simulink model "MCSI_simulation_2024_9_mod"  (R2021a)
settings: Solver=VariableStepAuto  StartTime=0.0  StopTime=5/cfg.fl  RelTol=1e-3
undefined symbols (not defined in the file or in its folder): cfg
libraries: spsIdealSwitchLib x54, spsSeriesRLCBranchLib x19, simulink x12, spsCurrentMeasurementLib x10, commutil2 x9, spsTriangleGeneratorLib x9, spsMeanLib x2, spsThreePhaseSeriesRLCBranchLib x2, spsThreePhaseVIMeasurementLib x2, spsControlledCurrentSourceLib x1, spsGroundLib x1, spsThreePhaseProgrammableGeneratorLib x1
settings Model: Creator=Damian  LastModifiedBy=Damian

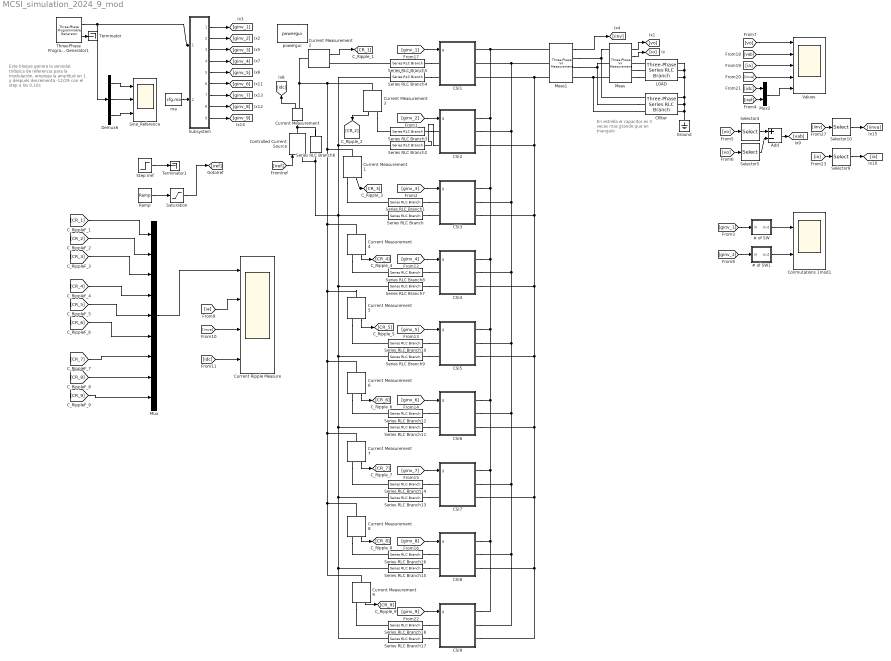
== system MCSI_simulation_2024_9_mod ==
  note: Este bloque genera la senoidal
      | trifásica de referencia para la
      | modulación, empieza la amplitud
      | en 1 y después decrementa -12/29
      | con el step a los 0.16s
  note: En estrella el capacitor
      | es 3 veces mas grande
      | que en triangulo
  # of SW : Subsystem
  # of SW1 : Subsystem
  Add : Sum  Inputs=+-
  CSI1 : Subsystem
  CSI2 : Subsystem
  CSI3 : Subsystem
  CSI4 : Subsystem
  CSI5 : Subsystem
  CSI6 : Subsystem
  CSI7 : Subsystem
  CSI8 : Subsystem
  CSI9 : Subsystem
  Cfilter : spsThreePhaseSeriesRLCBranchLib/Three-Phase Series RLC Branch  LConnTagsString=A|B|C  RConnTagsString=A|B|C  BranchType=C  Resistance=1  Inductance=cfg.c  Capacitance=cfg.c  Measurements=None
  Conmutations 1mod1 : Scope  NumInputPorts=2
  Controlled Current Source : spsControlledCurrentSourceLib/Controlled Current Source  Initialize=on  Source_Type=AC  Amplitude=0  Phase=0  Frequency=0  Measurements=None
  Current Measurement{,1..9} (10 alike) : spsCurrentMeasurementLib/Current Measurement  PhasorSimulation=off  OutputType=Complex  PSBequivalent=0
  Current Ripple Measure : Scope  NumInputPorts=4
  Demux6 : Demux  Outputs=3
  Ground : spsGroundLib/Ground  LConnTagsString=a
  LOAD : spsThreePhaseSeriesRLCBranchLib/Three-Phase Series RLC Branch  LConnTagsString=A|B|C  RConnTagsString=A|B|C  BranchType=RL  Resistance=cfg.r  Inductance=cfg.l  Capacitance=1e-6  Measurements=None
  Meas : spsThreePhaseVIMeasurementLib/Three-Phase V-I Measurement  VoltageMeasurement=phase-to-ground  SetLabelV=off  LabelV=Vabc  Vpu=off  VpuLL=off  CurrentMeasurement=yes  SetLabelI=off  LabelI=Iabc  Ipu=off  Pbase=100e6  Vbase=500e3  OutputType=Complex  PhasorSimulation=off  PSBequivalent=0
  Meas1 : spsThreePhaseVIMeasurementLib/Three-Phase V-I Measurement  VoltageMeasurement=no  SetLabelV=off  LabelV=Vabc  Vpu=off  VpuLL=off  CurrentMeasurement=yes  SetLabelI=off  LabelI=Iabc  Ipu=off  Pbase=100e6  Vbase=500e3  OutputType=Complex  PhasorSimulation=off  PSBequivalent=0
  Mux : Mux  Inputs=9
  Mux2 : Mux  Inputs=2
  Ramp : simulink/Sources/Ramp  slope=cfg.iref/cfg.cs_soft_start_time  start=0  InitialOutput=0
  Saturation : Saturate  UpperLimit=10  LowerLimit=0
  Selector10 : Selector  InputPortWidth=3  IndexOptions=Index vector (dialog)  Indices=1  OutputSizes=1
  Selector4 : Selector  InputPortWidth=3  IndexOptions=Index vector (dialog)  Indices=1  OutputSizes=1
  Selector5 : Selector  InputPortWidth=3  IndexOptions=Index vector (dialog)  Indices=2  OutputSizes=1
  Selector9 : Selector  InputPortWidth=3  IndexOptions=Index vector (dialog)  Indices=1  OutputSizes=1
  Series RLC Branch{,1..5,7..18} (18 alike) : spsSeriesRLCBranchLib/Series RLC Branch  LConnTagsString=__new0  RConnTagsString=__new0  BranchType=L  Resistance=1  Inductance=cfg.sharing_L  SetiL0=off  InitialCurrent=0  Capacitance=1e-6  Setx0=off  InitialVoltage=0  Measurements=None
  Series RLC Branch6 : spsSeriesRLCBranchLib/Series RLC Branch  LConnTagsString=__new0  RConnTagsString=__new0  BranchType=R  Resistance=1E5  Inductance=cfg.sharing_L  SetiL0=off  InitialCurrent=0  Capacitance=1e-6  Setx0=off  InitialVoltage=0  Measurements=None
  Sine_Reference : Scope  NumInputPorts=3
  Step Iref : Step  Time=12/cfg.fl  Before=cfg.iref  After=0.6*cfg.iref  SampleTime=cfg.ts
  Subsystem : Subsystem
  Terminator : Terminator
  Terminator1 : Terminator
  Three-Phase Programmable Generator1 : spsThreePhaseProgrammableGeneratorLib/Three-Phase Programmable Generator  Par_Vps=[1,-30, cfg.fl]  VariationEntity=None  VariationType=Step  VariationStep=-12/29  VariationRate=10  VariationMag=0.3  VariationFreq=2  Par_Timing_Variation="[8/cfg.fl  10]"  SinglePhase=on  Yampli=[1 0.2 1.2 1.0]  Xtime=[0 0.1 0.15 0.2]  HarmonicGeneration=off  Par_HarmoA="[3  5  -25 0]"  Par_HarmoB="[5  10  35  2]"  Par_Timing_Harmo="[ 0.05  99]"  Ts=cfg.ts
      settings: SourceProductBaseCode=PS
  Values : Scope  NumInputPorts=5
  ma : Constant  Value=cfg.ma
  powergui : spspowerguiLib/powergui  Priority=1  SimulationMode=Discrete  SampleTime=cfg.ts  frequency=60  Iterations=50  frequencyindice=0  Pbase=100e6  ErrMax=1e-4  UnitsV=kV  UnitsW=MW  buscounter=0  FunctionMessages=off  echomessages=off  EnableUseOfTLC=off  CurrentSourceSwitches=off  DisableSnubberDevices=off  DisableRonSwitches=off  DisableVfSwitches=off  DisplayEquations=off  AutomaticDiscreteSolvers=off  SolverType=Backward Euler  Interpol=off  ExternalGateDelay=off  methode=off  Ts=0  x0status=blocks  SPID=off  SwTol=0  HookPort=off  NonlinearTolerance=1e-4  nMaxIteration=100  ContinueOnMaxIteration=off  RestoreLinks=warning  ResistiveCurrentMeasurement=off  Frange=[0:2:500]  Ylog=off  Xlog=on  ShowGrid=off  save=off  variable=ZData  structure=one_mod_model  ZoomFFT=off  StartTime=0.12  cycles=1  DisplayStyle=1  fundamental=50  FreqAxis=off  MaxFrequency=1000  frequencyindicesteady=1  RmsSteady=1  display=off
  wires:
  [iref] -> Controlled Current Source/1
  Current Measurement/1 -> [idc]
  ma/1 -> Subsystem/2(ma)
  Three-Phase Programmable Generator1/2 -> Terminator/1
  Three-Phase Programmable Generator1/1 -> Subsystem/1(Vabc), Demux6/1
  Demux6/3 -> Sine_Reference/3
  Demux6/2 -> Sine_Reference/2
  Demux6/1 -> Sine_Reference/1
  [ginv_1] -> CSI1/1(g)
  Meas/1 -> [vo]
  Meas/2 -> [io]
  Meas1/1 -> [iinv]
  [iref] -> Mux2/2
  [idc] -> Mux2/1
  Mux2/1 -> Values/5
  [vo] -> Values/1
  [iinva] -> Values/4
  [ia] -> Values/3
  [vab] -> Values/2
  [vo] -> Selector4/1
  [vo] -> Selector5/1
  Selector4/1 -> Add/1
  Selector5/1 -> Add/2
  Add/1 -> [vab]
  [iinv] -> Selector10/1
  [io] -> Selector9/1
  Selector10/1 -> [iinva]
  Selector9/1 -> [ia]
  [ginv_2] -> CSI2/1(g)
  [ginv_3] -> CSI3/1(g)
  [ginv_1] -> # of SW/1(in)
  # of SW/1(out) -> Conmutations 1mod1/1
  # of SW1/1(out) -> Conmutations 1mod1/2
  [ginv_2] -> # of SW1/1(in)
  Saturation/1 -> [iref]
  Ramp/1 -> Saturation/1
  Step Iref/1 -> Terminator1/1
  Current Measurement2/1 -> [CR_1]
  Current Measurement3/1 -> [CR_2]
  Current Measurement1/1 -> [CR_3]
  [ia] -> Current Ripple Measure/2
  [iinva] -> Current Ripple Measure/3
  [idc] -> Current Ripple Measure/4
  [CR_1] -> Mux/1
  [CR_2] -> Mux/2
  [CR_3] -> Mux/3
  Mux/1 -> Current Ripple Measure/1
  Subsystem/1(g_1) -> [ginv_1]
  Subsystem/2(g_2) -> [ginv_2]
  Subsystem/3(g_3) -> [ginv_3]
  Subsystem/4(g_4) -> [ginv_4]
  Subsystem/5(g_5) -> [ginv_5]
  Subsystem/6(g_6) -> [ginv_6]
  Subsystem/7(g_7) -> [ginv_7]
  Subsystem/8(g_8) -> [ginv_8]
  Subsystem/9(g_9) -> [ginv_9]
  [ginv_4] -> CSI4/1(g)
  [ginv_5] -> CSI5/1(g)
  [ginv_6] -> CSI6/1(g)
  [ginv_7] -> CSI7/1(g)
  [ginv_8] -> CSI8/1(g)
  [ginv_9] -> CSI9/1(g)
  Current Measurement9/1 -> [CR_9]
  Current Measurement8/1 -> [CR_8]
  Current Measurement7/1 -> [CR_7]
  Current Measurement6/1 -> [CR_6]
  Current Measurement5/1 -> [CR_5]
  Current Measurement4/1 -> [CR_4]
  [CR_4] -> Mux/4
  [CR_5] -> Mux/5
  [CR_6] -> Mux/6
  [CR_7] -> Mux/7
  [CR_8] -> Mux/8
  [CR_9] -> Mux/9
  connections:
  Current Measurement/LConn1 -- Series RLC Branch6/LConn1 -- Controlled Current Source/RConn1
  Meas/LConn3 -- Cfilter/LConn3 -- Meas1/RConn3
  Meas/LConn1 -- Meas1/RConn1 -- Cfilter/LConn1
  LOAD/RConn2 -- LOAD/RConn1 -- LOAD/RConn3 -- Cfilter/RConn1 -- Cfilter/RConn2 -- Cfilter/RConn3 -- Ground/LConn1
  Cfilter/LConn2 -- Meas1/RConn2 -- Meas/LConn2
  LOAD/LConn1 -- Meas/RConn1
  Meas/RConn2 -- LOAD/LConn2
  Meas/RConn3 -- LOAD/LConn3
  Meas1/LConn1 -- CSI9/RConn1 -- CSI8/RConn1 -- CSI7/RConn1 -- CSI6/RConn1 -- CSI5/RConn1 -- CSI4/RConn1 -- CSI3/RConn1 -- CSI2/RConn1 -- CSI1/RConn1
  Meas1/LConn2 -- CSI9/RConn2 -- CSI8/RConn2 -- CSI7/RConn2 -- CSI6/RConn2 -- CSI5/RConn2 -- CSI4/RConn2 -- CSI3/RConn2 -- CSI2/RConn2 -- CSI1/RConn2
  Meas1/LConn3 -- CSI9/RConn3 -- CSI8/RConn3 -- CSI7/RConn3 -- CSI6/RConn3 -- CSI5/RConn3 -- CSI4/RConn3 -- CSI3/RConn3 -- CSI2/RConn3 -- CSI1/RConn3
  Series RLC Branch4/RConn1 -- CSI1/LConn2
  Series RLC Branch5/RConn1 -- CSI1/LConn1
  Series RLC Branch3/RConn1 -- CSI2/LConn2
  Series RLC Branch2/RConn1 -- CSI2/LConn1
  Series RLC Branch1/RConn1 -- CSI3/LConn1
  Series RLC Branch/RConn1 -- CSI3/LConn2
  Controlled Current Source/LConn1 -- Series RLC Branch17/LConn1 -- Series RLC Branch15/LConn1 -- Series RLC Branch13/LConn1 -- Series RLC Branch11/LConn1 -- Series RLC Branch9/LConn1 -- Series RLC Branch7/LConn1 -- Series RLC Branch2/LConn1 -- Series RLC Branch4/LConn1 -- Series RLC Branch/LConn1 -- Series RLC Branch6/RConn1
  Current Measurement3/RConn1 -- Series RLC Branch3/LConn1
  Current Measurement2/LConn1 -- Current Measurement1/LConn1 -- Current Measurement4/LConn1 -- Current Measurement5/LConn1 -- Current Measurement6/LConn1 -- Current Measurement7/LConn1 -- Current Measurement8/LConn1 -- Current Measurement9/LConn1 -- Current Measurement3/LConn1 -- Current Measurement/RConn1
  Current Measurement1/RConn1 -- Series RLC Branch1/LConn1
  Series RLC Branch5/LConn1 -- Current Measurement2/RConn1
  Series RLC Branch8/RConn1 -- CSI4/LConn1
  Series RLC Branch7/RConn1 -- CSI4/LConn2
  Series RLC Branch10/RConn1 -- CSI5/LConn1
  Series RLC Branch9/RConn1 -- CSI5/LConn2
  Series RLC Branch12/RConn1 -- CSI6/LConn1
  Series RLC Branch11/RConn1 -- CSI6/LConn2
  Series RLC Branch14/RConn1 -- CSI7/LConn1
  Series RLC Branch13/RConn1 -- CSI7/LConn2
  Series RLC Branch16/RConn1 -- CSI8/LConn1
  Series RLC Branch15/RConn1 -- CSI8/LConn2
  Series RLC Branch18/RConn1 -- CSI9/LConn1
  Series RLC Branch17/RConn1 -- CSI9/LConn2
  Current Measurement9/RConn1 -- Series RLC Branch18/LConn1
  Current Measurement8/RConn1 -- Series RLC Branch16/LConn1
  Current Measurement7/RConn1 -- Series RLC Branch14/LConn1
  Current Measurement6/RConn1 -- Series RLC Branch12/LConn1
  Current Measurement5/RConn1 -- Series RLC Branch10/LConn1
  Current Measurement4/RConn1 -- Series RLC Branch8/LConn1

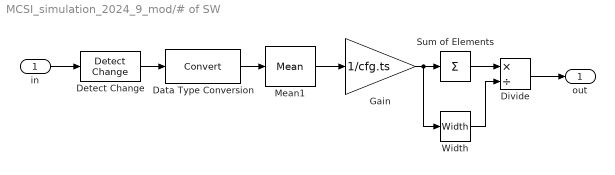
== system MCSI_simulation_2024_9_mod/# of SW ==
  in : Inport
  Data Type Conversion : DataTypeConversion
  Detect Change : simulink/Logic and Bit Operations/Detect Change  vinit=0  OutDataTypeStr=boolean
  Divide : Product  Inputs=*/
  Gain : Gain  Gain=1/cfg.ts
  Mean1 : spsMeanLib/Mean  Freq=cfg.fl  Vinit=0  Ts=cfg.ts
  Sum of Elements : Sum  Inputs=+
  Width : Width
  out : Outport
  wires:
  Detect Change/1 -> Data Type Conversion/1
  Mean1/1 -> Gain/1
  Data Type Conversion/1 -> Mean1/1
  in/1 -> Detect Change/1
  Gain/1 -> Width/1, Sum of Elements/1
  Sum of Elements/1 -> Divide/1
  Width/1 -> Divide/2
  Divide/1 -> out/1

== system MCSI_simulation_2024_9_mod/# of SW1 ==
  in : Inport
  Data Type Conversion : DataTypeConversion
  Detect Change : simulink/Logic and Bit Operations/Detect Change  vinit=0  OutDataTypeStr=boolean
  Gain : Gain  Gain=1/cfg.ts
  Mean1 : spsMeanLib/Mean  Freq=cfg.fl  Vinit=0  Ts=cfg.ts
  out : Outport
  wires:
  Detect Change/1 -> Data Type Conversion/1
  Mean1/1 -> Gain/1
  Data Type Conversion/1 -> Mean1/1
  in/1 -> Detect Change/1
  Gain/1 -> out/1

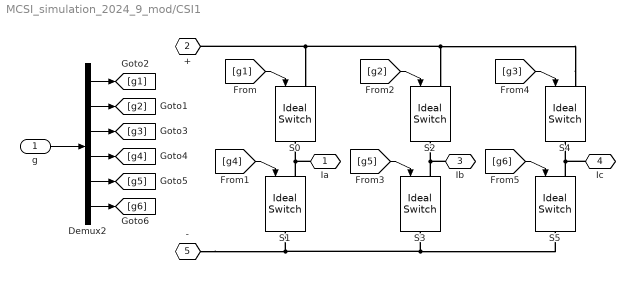
== system MCSI_simulation_2024_9_mod/CSI1 ==
  g : Inport
  Demux2 : Demux  Outputs=6
  S{0..5} (6 alike) : spsIdealSwitchLib/Ideal Switch  Ron=cfg.switch.Ron  Lon=0  IC=0  Rs=cfg.switch.snubber_Rs  Cs=cfg.switch.snubber_Cs  Measurements=off
  Ia : PMIOPort  Side=Right
  + : PMIOPort  Port=2  Side=Left
  Ib : PMIOPort  Port=3  Side=Right
  Ic : PMIOPort  Port=4  Side=Right
  - : PMIOPort  Port=5  Side=Left
  wires:
  Demux2/1 -> [g1]
  Demux2/4 -> [g4]
  g/1 -> Demux2/1
  [g4] -> S1/1
  [g2] -> S2/1
  [g5] -> S3/1
  Demux2/5 -> [g5]
  [g3] -> S4/1
  [g6] -> S5/1
  Demux2/6 -> [g6]
  Demux2/3 -> [g3]
  Demux2/2 -> [g2]
  [g1] -> S0/1
  connections:
  S1/LConn1 -- Ia/RConn1 -- S0/RConn1
  S3/LConn1 -- Ib/RConn1 -- S2/RConn1
  S5/LConn1 -- Ic/RConn1 -- S4/RConn1
  S4/LConn1 -- S2/LConn1 -- S0/LConn1 -- +/RConn1
  -/RConn1 -- S5/RConn1 -- S3/RConn1 -- S1/RConn1

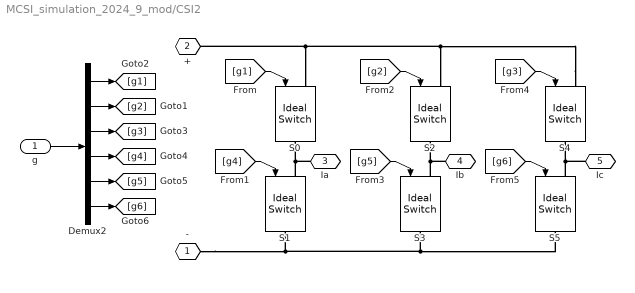
== system MCSI_simulation_2024_9_mod/CSI2 ==
  g : Inport
  Demux2 : Demux  Outputs=6
  S{0..5} (6 alike) : spsIdealSwitchLib/Ideal Switch  Ron=cfg.switch.Ron  Lon=0  IC=0  Rs=cfg.switch.snubber_Rs  Cs=cfg.switch.snubber_Cs  Measurements=off
  - : PMIOPort  Side=Left
  + : PMIOPort  Port=2  Side=Left
  Ia : PMIOPort  Port=3  Side=Right
  Ib : PMIOPort  Port=4  Side=Right
  Ic : PMIOPort  Port=5  Side=Right
  wires:
  Demux2/1 -> [g1]
  Demux2/4 -> [g4]
  g/1 -> Demux2/1
  [g4] -> S1/1
  [g2] -> S2/1
  [g5] -> S3/1
  Demux2/5 -> [g5]
  [g3] -> S4/1
  [g6] -> S5/1
  Demux2/6 -> [g6]
  Demux2/3 -> [g3]
  Demux2/2 -> [g2]
  [g1] -> S0/1
  connections:
  S1/LConn1 -- Ia/RConn1 -- S0/RConn1
  S3/LConn1 -- Ib/RConn1 -- S2/RConn1
  S5/LConn1 -- Ic/RConn1 -- S4/RConn1
  S4/LConn1 -- S2/LConn1 -- S0/LConn1 -- +/RConn1
  -/RConn1 -- S5/RConn1 -- S3/RConn1 -- S1/RConn1

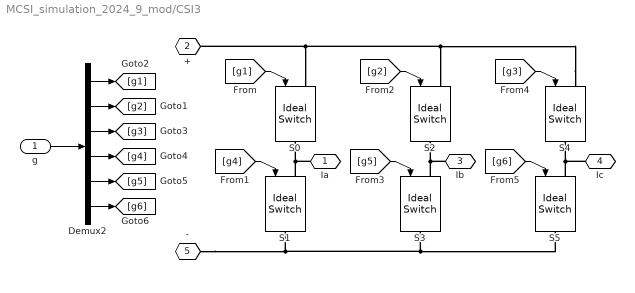
== system MCSI_simulation_2024_9_mod/CSI3 ==
  g : Inport
  Demux2 : Demux  Outputs=6
  S{0..5} (6 alike) : spsIdealSwitchLib/Ideal Switch  Ron=cfg.switch.Ron  Lon=0  IC=0  Rs=cfg.switch.snubber_Rs  Cs=cfg.switch.snubber_Cs  Measurements=off
  Ia : PMIOPort  Side=Right
  + : PMIOPort  Port=2  Side=Left
  Ib : PMIOPort  Port=3  Side=Right
  Ic : PMIOPort  Port=4  Side=Right
  - : PMIOPort  Port=5  Side=Left
  wires:
  Demux2/1 -> [g1]
  Demux2/4 -> [g4]
  g/1 -> Demux2/1
  [g4] -> S1/1
  [g2] -> S2/1
  [g5] -> S3/1
  Demux2/5 -> [g5]
  [g3] -> S4/1
  [g6] -> S5/1
  Demux2/6 -> [g6]
  Demux2/3 -> [g3]
  Demux2/2 -> [g2]
  [g1] -> S0/1
  connections:
  S1/LConn1 -- Ia/RConn1 -- S0/RConn1
  S3/LConn1 -- Ib/RConn1 -- S2/RConn1
  S5/LConn1 -- Ic/RConn1 -- S4/RConn1
  S4/LConn1 -- S2/LConn1 -- S0/LConn1 -- +/RConn1
  -/RConn1 -- S5/RConn1 -- S3/RConn1 -- S1/RConn1

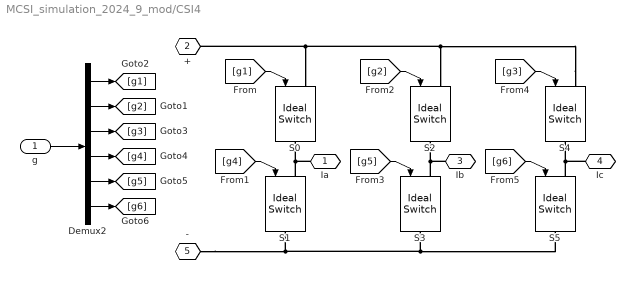
== system MCSI_simulation_2024_9_mod/CSI4 ==
  g : Inport
  Demux2 : Demux  Outputs=6
  S{0..5} (6 alike) : spsIdealSwitchLib/Ideal Switch  Ron=cfg.switch.Ron  Lon=0  IC=0  Rs=cfg.switch.snubber_Rs  Cs=cfg.switch.snubber_Cs  Measurements=off
  Ia : PMIOPort  Side=Right
  + : PMIOPort  Port=2  Side=Left
  Ib : PMIOPort  Port=3  Side=Right
  Ic : PMIOPort  Port=4  Side=Right
  - : PMIOPort  Port=5  Side=Left
  wires:
  Demux2/1 -> [g1]
  Demux2/4 -> [g4]
  g/1 -> Demux2/1
  [g4] -> S1/1
  [g2] -> S2/1
  [g5] -> S3/1
  Demux2/5 -> [g5]
  [g3] -> S4/1
  [g6] -> S5/1
  Demux2/6 -> [g6]
  Demux2/3 -> [g3]
  Demux2/2 -> [g2]
  [g1] -> S0/1
  connections:
  S1/LConn1 -- Ia/RConn1 -- S0/RConn1
  S3/LConn1 -- Ib/RConn1 -- S2/RConn1
  S5/LConn1 -- Ic/RConn1 -- S4/RConn1
  S4/LConn1 -- S2/LConn1 -- S0/LConn1 -- +/RConn1
  -/RConn1 -- S5/RConn1 -- S3/RConn1 -- S1/RConn1

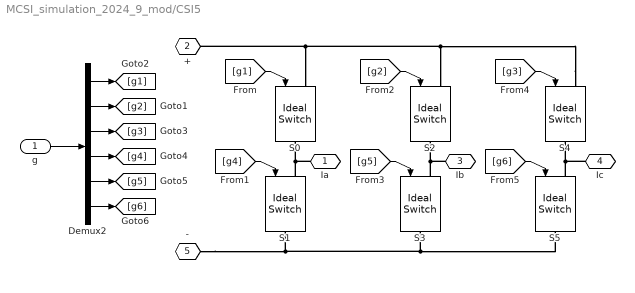
== system MCSI_simulation_2024_9_mod/CSI5 ==
  g : Inport
  Demux2 : Demux  Outputs=6
  S{0..5} (6 alike) : spsIdealSwitchLib/Ideal Switch  Ron=cfg.switch.Ron  Lon=0  IC=0  Rs=cfg.switch.snubber_Rs  Cs=cfg.switch.snubber_Cs  Measurements=off
  Ia : PMIOPort  Side=Right
  + : PMIOPort  Port=2  Side=Left
  Ib : PMIOPort  Port=3  Side=Right
  Ic : PMIOPort  Port=4  Side=Right
  - : PMIOPort  Port=5  Side=Left
  wires:
  Demux2/1 -> [g1]
  Demux2/4 -> [g4]
  g/1 -> Demux2/1
  [g4] -> S1/1
  [g2] -> S2/1
  [g5] -> S3/1
  Demux2/5 -> [g5]
  [g3] -> S4/1
  [g6] -> S5/1
  Demux2/6 -> [g6]
  Demux2/3 -> [g3]
  Demux2/2 -> [g2]
  [g1] -> S0/1
  connections:
  S1/LConn1 -- Ia/RConn1 -- S0/RConn1
  S3/LConn1 -- Ib/RConn1 -- S2/RConn1
  S5/LConn1 -- Ic/RConn1 -- S4/RConn1
  S4/LConn1 -- S2/LConn1 -- S0/LConn1 -- +/RConn1
  -/RConn1 -- S5/RConn1 -- S3/RConn1 -- S1/RConn1

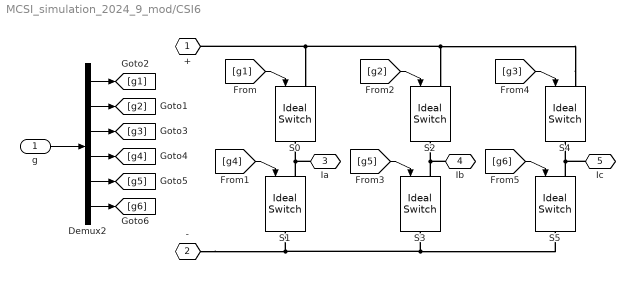
== system MCSI_simulation_2024_9_mod/CSI6 ==
  g : Inport
  Demux2 : Demux  Outputs=6
  S{0..5} (6 alike) : spsIdealSwitchLib/Ideal Switch  Ron=cfg.switch.Ron  Lon=0  IC=0  Rs=cfg.switch.snubber_Rs  Cs=cfg.switch.snubber_Cs  Measurements=off
  + : PMIOPort  Side=Left
  - : PMIOPort  Port=2  Side=Left
  Ia : PMIOPort  Port=3  Side=Right
  Ib : PMIOPort  Port=4  Side=Right
  Ic : PMIOPort  Port=5  Side=Right
  wires:
  Demux2/1 -> [g1]
  Demux2/4 -> [g4]
  g/1 -> Demux2/1
  [g4] -> S1/1
  [g2] -> S2/1
  [g5] -> S3/1
  Demux2/5 -> [g5]
  [g3] -> S4/1
  [g6] -> S5/1
  Demux2/6 -> [g6]
  Demux2/3 -> [g3]
  Demux2/2 -> [g2]
  [g1] -> S0/1
  connections:
  S1/LConn1 -- Ia/RConn1 -- S0/RConn1
  S3/LConn1 -- Ib/RConn1 -- S2/RConn1
  S5/LConn1 -- Ic/RConn1 -- S4/RConn1
  S4/LConn1 -- S2/LConn1 -- S0/LConn1 -- +/RConn1
  -/RConn1 -- S5/RConn1 -- S3/RConn1 -- S1/RConn1

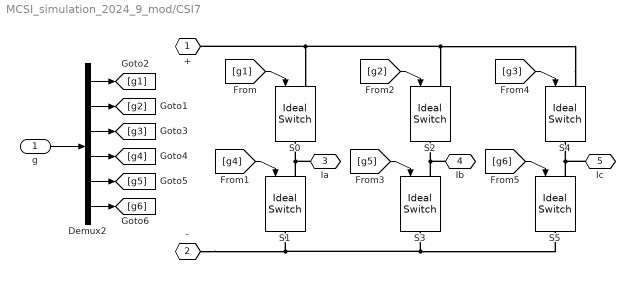
== system MCSI_simulation_2024_9_mod/CSI7 ==
  g : Inport
  Demux2 : Demux  Outputs=6
  S{0..5} (6 alike) : spsIdealSwitchLib/Ideal Switch  Ron=cfg.switch.Ron  Lon=0  IC=0  Rs=cfg.switch.snubber_Rs  Cs=cfg.switch.snubber_Cs  Measurements=off
  + : PMIOPort  Side=Left
  - : PMIOPort  Port=2  Side=Left
  Ia : PMIOPort  Port=3  Side=Right
  Ib : PMIOPort  Port=4  Side=Right
  Ic : PMIOPort  Port=5  Side=Right
  wires:
  Demux2/1 -> [g1]
  Demux2/4 -> [g4]
  g/1 -> Demux2/1
  [g4] -> S1/1
  [g2] -> S2/1
  [g5] -> S3/1
  Demux2/5 -> [g5]
  [g3] -> S4/1
  [g6] -> S5/1
  Demux2/6 -> [g6]
  Demux2/3 -> [g3]
  Demux2/2 -> [g2]
  [g1] -> S0/1
  connections:
  S1/LConn1 -- Ia/RConn1 -- S0/RConn1
  S3/LConn1 -- Ib/RConn1 -- S2/RConn1
  S5/LConn1 -- Ic/RConn1 -- S4/RConn1
  S4/LConn1 -- S2/LConn1 -- S0/LConn1 -- +/RConn1
  -/RConn1 -- S5/RConn1 -- S3/RConn1 -- S1/RConn1

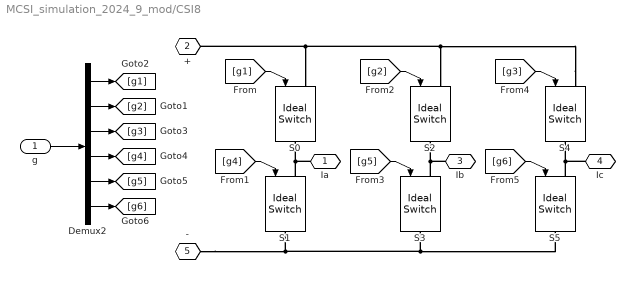
== system MCSI_simulation_2024_9_mod/CSI8 ==
  g : Inport
  Demux2 : Demux  Outputs=6
  S{0..5} (6 alike) : spsIdealSwitchLib/Ideal Switch  Ron=cfg.switch.Ron  Lon=0  IC=0  Rs=cfg.switch.snubber_Rs  Cs=cfg.switch.snubber_Cs  Measurements=off
  Ia : PMIOPort  Side=Right
  + : PMIOPort  Port=2  Side=Left
  Ib : PMIOPort  Port=3  Side=Right
  Ic : PMIOPort  Port=4  Side=Right
  - : PMIOPort  Port=5  Side=Left
  wires:
  Demux2/1 -> [g1]
  Demux2/4 -> [g4]
  g/1 -> Demux2/1
  [g4] -> S1/1
  [g2] -> S2/1
  [g5] -> S3/1
  Demux2/5 -> [g5]
  [g3] -> S4/1
  [g6] -> S5/1
  Demux2/6 -> [g6]
  Demux2/3 -> [g3]
  Demux2/2 -> [g2]
  [g1] -> S0/1
  connections:
  S1/LConn1 -- Ia/RConn1 -- S0/RConn1
  S3/LConn1 -- Ib/RConn1 -- S2/RConn1
  S5/LConn1 -- Ic/RConn1 -- S4/RConn1
  S4/LConn1 -- S2/LConn1 -- S0/LConn1 -- +/RConn1
  -/RConn1 -- S5/RConn1 -- S3/RConn1 -- S1/RConn1

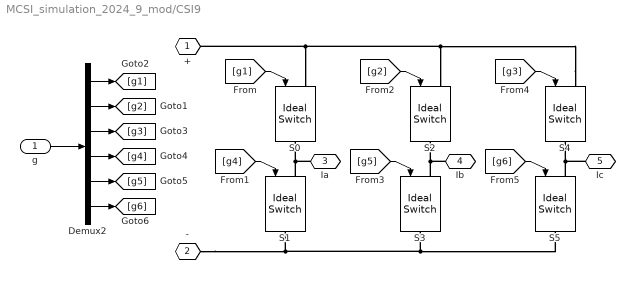
== system MCSI_simulation_2024_9_mod/CSI9 ==
  g : Inport
  Demux2 : Demux  Outputs=6
  S{0..5} (6 alike) : spsIdealSwitchLib/Ideal Switch  Ron=cfg.switch.Ron  Lon=0  IC=0  Rs=cfg.switch.snubber_Rs  Cs=cfg.switch.snubber_Cs  Measurements=off
  + : PMIOPort  Side=Left
  - : PMIOPort  Port=2  Side=Left
  Ia : PMIOPort  Port=3  Side=Right
  Ib : PMIOPort  Port=4  Side=Right
  Ic : PMIOPort  Port=5  Side=Right
  wires:
  Demux2/1 -> [g1]
  Demux2/4 -> [g4]
  g/1 -> Demux2/1
  [g4] -> S1/1
  [g2] -> S2/1
  [g5] -> S3/1
  Demux2/5 -> [g5]
  [g3] -> S4/1
  [g6] -> S5/1
  Demux2/6 -> [g6]
  Demux2/3 -> [g3]
  Demux2/2 -> [g2]
  [g1] -> S0/1
  connections:
  S1/LConn1 -- Ia/RConn1 -- S0/RConn1
  S3/LConn1 -- Ib/RConn1 -- S2/RConn1
  S5/LConn1 -- Ic/RConn1 -- S4/RConn1
  S4/LConn1 -- S2/LConn1 -- S0/LConn1 -- +/RConn1
  -/RConn1 -- S5/RConn1 -- S3/RConn1 -- S1/RConn1

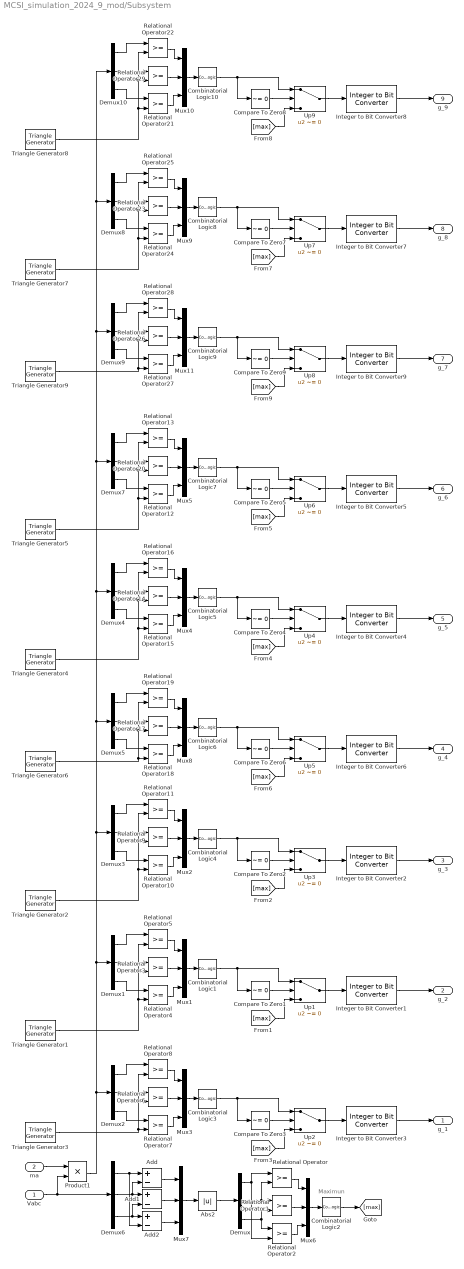
== system MCSI_simulation_2024_9_mod/Subsystem ==
  note: Maximun
  Vabc : Inport
  ma : Inport  Port=2
  Abs2 : Abs
  Add : Sum  Inputs=+-
  Add1 : Sum  Inputs=+-
  Add2 : Sum  Inputs=+-
  Combinatorial Logic{1,3..10} (9 alike) : CombinatorialLogic  TruthTable=bin2dec(['000000'; '001010'; '010100'; '001100'; '100001'; '100010'; '010001'; '000000'])
  Combinatorial Logic2 : CombinatorialLogic  TruthTable=bin2dec(['111111'; '001001'; '010010'; '010010'; '100100'; '001001'; '100100'; '111111'])
  Compare To Zero{1..9} (9 alike) : simulink/Logic and Bit Operations/Compare To Zero  relop=~=  OutDataTypeStr=boolean
  Demux{,1..10} (11 alike) : Demux  Outputs=3
  Integer to Bit Converter{1..9} (9 alike) : commutil2/Integer to Bit Converter  nbits=6  signedInputValues=Unsigned  bitOrder=MSB first  outDtype=Inherit via internal rule
  Mux{1..11} (11 alike) : Mux  Inputs=3
  Product1 : Product
  Relational Operator{,1..29} (30 alike) : RelationalOperator  OutDataTypeStr=boolean  RndMeth=Nearest
  Triangle Generator1 : spsTriangleGeneratorLib/Triangle Generator  Freq=cfg.fl*cfg.mf  Phase=1*cfg.tri_phase_shift  Ts=cfg.ts
  Triangle Generator2 : spsTriangleGeneratorLib/Triangle Generator  Freq=cfg.fl*cfg.mf  Phase=2*cfg.tri_phase_shift  Ts=cfg.ts
  Triangle Generator3 : spsTriangleGeneratorLib/Triangle Generator  Freq=cfg.fl*cfg.mf  Phase=0  Ts=cfg.ts
  Triangle Generator4 : spsTriangleGeneratorLib/Triangle Generator  Freq=cfg.fl*cfg.mf  Phase=4*cfg.tri_phase_shift  Ts=cfg.ts
  Triangle Generator5 : spsTriangleGeneratorLib/Triangle Generator  Freq=cfg.fl*cfg.mf  Phase=5*cfg.tri_phase_shift  Ts=cfg.ts
  Triangle Generator6 : spsTriangleGeneratorLib/Triangle Generator  Freq=cfg.fl*cfg.mf  Phase=3*cfg.tri_phase_shift  Ts=cfg.ts
  Triangle Generator7 : spsTriangleGeneratorLib/Triangle Generator  Freq=cfg.fl*cfg.mf  Phase=7*cfg.tri_phase_shift  Ts=cfg.ts
  Triangle Generator8 : spsTriangleGeneratorLib/Triangle Generator  Freq=cfg.fl*cfg.mf  Phase=8*cfg.tri_phase_shift  Ts=cfg.ts
  Triangle Generator9 : spsTriangleGeneratorLib/Triangle Generator  Freq=cfg.fl*cfg.mf  Phase=6*cfg.tri_phase_shift  Ts=cfg.ts
  Up{1..9} (9 alike) : Switch  Criteria=u2 ~= 0
  g_1 : Outport
  g_2 : Outport  Port=2
  g_3 : Outport  Port=3
  g_4 : Outport  Port=4
  g_5 : Outport  Port=5
  g_6 : Outport  Port=6
  g_7 : Outport  Port=7
  g_8 : Outport  Port=8
  g_9 : Outport  Port=9
  wires:
  Relational Operator/1 -> Mux6/1
  Demux/3 -> Relational Operator1/2, Relational Operator2/1
  Relational Operator1/1 -> Mux6/2
  Demux/2 -> Relational Operator/2, Relational Operator1/1
  Mux6/1 -> Combinatorial Logic2/1
  Relational Operator2/1 -> Mux6/3
  Vabc/1 -> Product1/2, Demux6/1
  Demux/1 -> Relational Operator/1, Relational Operator2/2
  Demux6/1 -> Add2/2, Add/1
  Demux6/2 -> Add/2, Add1/1
  Demux6/3 -> Add1/2, Add2/1
  Add/1 -> Mux7/1
  Add1/1 -> Mux7/2
  Add2/1 -> Mux7/3
  Abs2/1 -> Demux/1
  Mux7/1 -> Abs2/1
  Combinatorial Logic2/1 -> [max]
  ma/1 -> Product1/1
  Relational Operator7/1 -> Mux3/3
  Relational Operator8/1 -> Mux3/1
  Relational Operator6/1 -> Mux3/2
  Mux3/1 -> Combinatorial Logic3/1
  Combinatorial Logic3/1 -> Up2/1, Compare To Zero3/1
  Compare To Zero3/1 -> Up2/2
  Up2/1 -> Integer to Bit Converter3/1
  [max] -> Up2/3
  Triangle Generator3/1 -> Relational Operator8/2, Relational Operator6/2, Relational Operator7/2
  Demux2/3 -> Relational Operator7/1
  Demux2/2 -> Relational Operator6/1
  Demux2/1 -> Relational Operator8/1
  Integer to Bit Converter3/1 -> g_1/1
  Integer to Bit Converter1/1 -> g_2/1
  Relational Operator5/1 -> Mux1/1
  Demux1/1 -> Relational Operator5/1
  Mux1/1 -> Combinatorial Logic1/1
  Relational Operator3/1 -> Mux1/2
  [max] -> Up1/3
  Combinatorial Logic1/1 -> Up1/1, Compare To Zero1/1
  Demux1/2 -> Relational Operator3/1
  Up1/1 -> Integer to Bit Converter1/1
  Demux1/3 -> Relational Operator4/1
  Relational Operator4/1 -> Mux1/3
  Triangle Generator1/1 -> Relational Operator5/2, Relational Operator3/2, Relational Operator4/2
  Compare To Zero1/1 -> Up1/2
  Compare To Zero2/1 -> Up3/2
  Up3/1 -> Integer to Bit Converter2/1
  Relational Operator10/1 -> Mux2/3
  Demux3/2 -> Relational Operator9/1
  Demux3/3 -> Relational Operator10/1
  Relational Operator9/1 -> Mux2/2
  [max] -> Up3/3
  Demux3/1 -> Relational Operator11/1
  Combinatorial Logic4/1 -> Up3/1, Compare To Zero2/1
  Integer to Bit Converter2/1 -> g_3/1
  Relational Operator11/1 -> Mux2/1
  Triangle Generator2/1 -> Relational Operator11/2, Relational Operator9/2, Relational Operator10/2
  Mux2/1 -> Combinatorial Logic4/1
  Relational Operator13/1 -> Mux5/1
  Mux4/1 -> Combinatorial Logic5/1
  Integer to Bit Converter5/1 -> g_6/1
  Compare To Zero4/1 -> Up4/2
  Demux4/3 -> Relational Operator15/1
  Demux7/1 -> Relational Operator13/1
  Relational Operator15/1 -> Mux4/3
  Demux7/3 -> Relational Operator12/1
  [max] -> Up4/3
  Triangle Generator4/1 -> Relational Operator16/2, Relational Operator14/2, Relational Operator15/2
  Relational Operator20/1 -> Mux5/2
  Triangle Generator5/1 -> Relational Operator13/2, Relational Operator20/2, Relational Operator12/2
  Triangle Generator6/1 -> Relational Operator19/2, Relational Operator17/2, Relational Operator18/2
  Relational Operator19/1 -> Mux8/1
  Combinatorial Logic7/1 -> Up6/1, Compare To Zero5/1
  Combinatorial Logic6/1 -> Up5/1, Compare To Zero6/1
  Mux5/1 -> Combinatorial Logic7/1
  Mux8/1 -> Combinatorial Logic6/1
  [max] -> Up5/3
  Up5/1 -> Integer to Bit Converter6/1
  Demux7/2 -> Relational Operator20/1
  Integer to Bit Converter6/1 -> g_4/1
  Combinatorial Logic5/1 -> Up4/1, Compare To Zero4/1
  Compare To Zero5/1 -> Up6/2
  Up4/1 -> Integer to Bit Converter4/1
  Compare To Zero6/1 -> Up5/2
  Demux4/2 -> Relational Operator14/1
  Relational Operator14/1 -> Mux4/2
  [max] -> Up6/3
  Demux4/1 -> Relational Operator16/1
  Integer to Bit Converter4/1 -> g_5/1
  Relational Operator16/1 -> Mux4/1
  Demux5/1 -> Relational Operator19/1
  Demux5/2 -> Relational Operator17/1
  Relational Operator18/1 -> Mux8/3
  Relational Operator12/1 -> Mux5/3
  Demux5/3 -> Relational Operator18/1
  Relational Operator17/1 -> Mux8/2
  Up6/1 -> Integer to Bit Converter5/1
  Relational Operator22/1 -> Mux10/1
  Mux9/1 -> Combinatorial Logic8/1
  Integer to Bit Converter8/1 -> g_9/1
  Compare To Zero7/1 -> Up7/2
  Demux8/3 -> Relational Operator24/1
  Demux10/1 -> Relational Operator22/1
  Relational Operator24/1 -> Mux9/3
  Demux10/3 -> Relational Operator21/1
  [max] -> Up7/3
  Triangle Generator7/1 -> Relational Operator25/2, Relational Operator23/2, Relational Operator24/2
  Relational Operator29/1 -> Mux10/2
  Triangle Generator8/1 -> Relational Operator22/2, Relational Operator29/2, Relational Operator21/2
  Triangle Generator9/1 -> Relational Operator28/2, Relational Operator26/2, Relational Operator27/2
  Relational Operator28/1 -> Mux11/1
  Combinatorial Logic10/1 -> Up9/1, Compare To Zero8/1
  Combinatorial Logic9/1 -> Up8/1, Compare To Zero9/1
  Mux10/1 -> Combinatorial Logic10/1
  Mux11/1 -> Combinatorial Logic9/1
  [max] -> Up8/3
  Up8/1 -> Integer to Bit Converter9/1
  Demux10/2 -> Relational Operator29/1
  Product1/1 -> Demux10/1, Demux8/1, Demux9/1, Demux7/1, Demux4/1, Demux5/1, Demux3/1, Demux1/1, Demux2/1
  Integer to Bit Converter9/1 -> g_7/1
  Combinatorial Logic8/1 -> Up7/1, Compare To Zero7/1
  Compare To Zero8/1 -> Up9/2
  Up7/1 -> Integer to Bit Converter7/1
  Compare To Zero9/1 -> Up8/2
  Demux8/2 -> Relational Operator23/1
  Relational Operator23/1 -> Mux9/2
  [max] -> Up9/3
  Demux8/1 -> Relational Operator25/1
  Integer to Bit Converter7/1 -> g_8/1
  Relational Operator25/1 -> Mux9/1
  Demux9/1 -> Relational Operator28/1
  Demux9/2 -> Relational Operator26/1
  Relational Operator27/1 -> Mux11/3
  Relational Operator21/1 -> Mux10/3
  Demux9/3 -> Relational Operator27/1
  Relational Operator26/1 -> Mux11/2
  Up9/1 -> Integer to Bit Converter8/1
